simulink library "dbt"  (Simulink 8.1)
settings: Solver=ode1  StartTime=0.0  StopTime=Inf  FixedStep=0.001  RelTol=1e-3
PostLoadFcn:
  | , if any(exist('dsrtsu_mdlpostloadfcn', 'file') == [2, 3, 6]), try dsrtsu_mdlpostloadfcn('Execute', bdroot); catch fprintf('Error in PostLoadFcn (dsrtsu_mdlpostloadfcn) for model "%s":\n %s\n', bdroot, lasterr); end, end,
undefined symbols (not defined in the file or in its folder): AACC_VehSpdError_kph, KACC_ACCShortSetTimeGap_s, KACC_TGapTBAddedDecel_mps2, MACC_ACCFMTBLookUpDecel_mps2, MACC_ACCTBLookUpDecel_mps2, ZERO_FLOAT
libraries: hcu_lib x2
settings Model: DSRTSU_INTERNAL_RTI_VER=450  DSRTSU_INTERNAL_RTI_TYPE=rti1401  Creator=AT015555  LastModifiedBy=AT015555

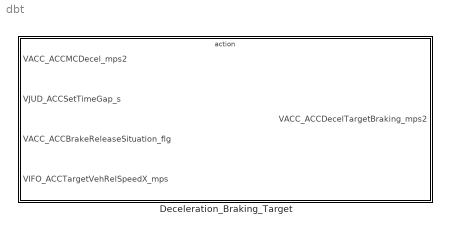
== system dbt ==
  Deceleration_Braking_Target : Subsystem  TreatAsAtomicUnit=on

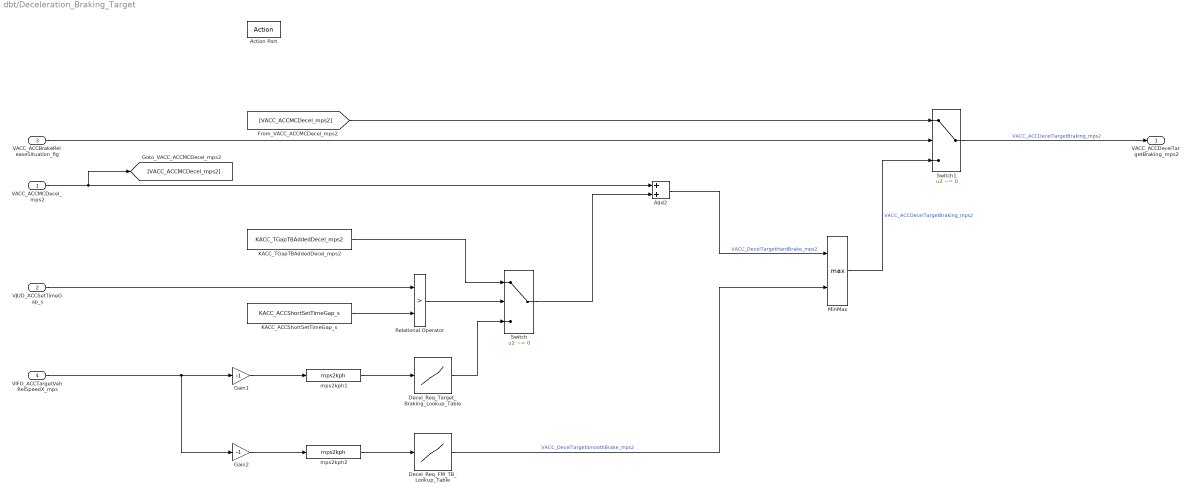
== system dbt/Deceleration_Braking_Target ==
  VACC_ACCMCDecel_mps2 : Inport
  VJUD_ACCSetTimeGap_s : Inport  Port=2
  VACC_ACCBrakeReleaseSituation_flg : Inport  Port=3
  VIFO_ACCTargetVehRelSpeedX_mps : Inport  Port=4
  Action Port : ActionPort
  Add2 : Sum
  Decel_Req_FM_TB_Lookup_Table : Lookup_n-D  NumberOfTableDimensions=1  BreakpointsForDimension1=AACC_VehSpdError_kph  Table=MACC_ACCFMTBLookUpDecel_mps2  ExtrapMethod=Clip  UseLastTableValue=on  RndMeth=Simplest  InputSameDT=on
  Decel_Req_Target_Braking_Lookup_Table : Lookup_n-D  NumberOfTableDimensions=1  BreakpointsForDimension1=AACC_VehSpdError_kph  Table=MACC_ACCTBLookUpDecel_mps2  ExtrapMethod=Clip  UseLastTableValue=on  RndMeth=Simplest  InputSameDT=on
  Gain1 : Gain  Gain=-1
  Gain2 : Gain  Gain=-1
  KACC_ACCShortSetTimeGap_s : Constant  Value=KACC_ACCShortSetTimeGap_s
  KACC_TGapTBAddedDecel_mps2 : Constant  Value=KACC_TGapTBAddedDecel_mps2
  MinMax : MinMax  Function=max  Inputs=2
  Relational Operator : RelationalOperator  Operator=>  OutDataTypeStr=boolean
  Switch : Switch  Criteria=u2 ~= 0
  Switch1 : Switch  Criteria=u2 ~= 0
  mps2kph1 : hcu_lib/mps2kph
  mps2kph2 : hcu_lib/mps2kph
  VACC_ACCDecelTargetBraking_mps2 : Outport  OutputWhenDisabled=reset  InitialOutput=ZERO_FLOAT
  wires:
  Gain1/1 -> mps2kph1/1
  mps2kph1/1 -> Decel_Req_Target_Braking_Lookup_Table/1
  VACC_ACCMCDecel_mps2/1 -> Add2/1, [VACC_ACCMCDecel_mps2]
  Decel_Req_Target_Braking_Lookup_Table/1 -> Switch/3
  mps2kph2/1 -> Decel_Req_FM_TB_Lookup_Table/1
  Gain2/1 -> mps2kph2/1
  VIFO_ACCTargetVehRelSpeedX_mps/1 -> Gain2/1, Gain1/1
  Add2/1 -> MinMax/1  "VACC_DecelTargetHardBrake_mps2"
  Decel_Req_FM_TB_Lookup_Table/1 -> MinMax/2  "VACC_DecelTargetSmoothBrake_mps2"
  Switch1/1 -> VACC_ACCDecelTargetBraking_mps2/1  "VACC_ACCDecelTargetBraking_mps2"
  KACC_ACCShortSetTimeGap_s/1 -> Relational Operator/2
  VJUD_ACCSetTimeGap_s/1 -> Relational Operator/1
  Relational Operator/1 -> Switch/2
  KACC_TGapTBAddedDecel_mps2/1 -> Switch/1
  Switch/1 -> Add2/2
  VACC_ACCBrakeReleaseSituation_flg/1 -> Switch1/2
  [VACC_ACCMCDecel_mps2] -> Switch1/1
  MinMax/1 -> Switch1/3  "VACC_ACCDecelTargetBraking_mps2"
